simulink model "Forced_SMD_System"  (R2023b)
settings: Solver=VariableStepAuto  StartTime=0.0  StopTime=5  MaxStep=0.01  RelTol=1e-3
model workspace (MAT data in the model file):
  b = 0.5
  k = 1
  m = 10
settings Model: Creator=91839  LastModifiedBy=siva kumar
settings SolverCC: AlgebraicLoopSolver=TrustRegion
settings DataIOCC: ExternalInput=data  SaveFormat=Array  DSMLogging=off  ReturnWorkspaceOutputs=off
settings DebuggingCC: UnconnectedInputMsg=warning  UnconnectedOutputMsg=warning  UnconnectedLineMsg=warning
settings ModelReferenceCC: EnableRefExpFcnMdlSchedulingChecks=on
settings SFSimCC: CustomCodeUndefinedFunction=UseInterfaceOnly

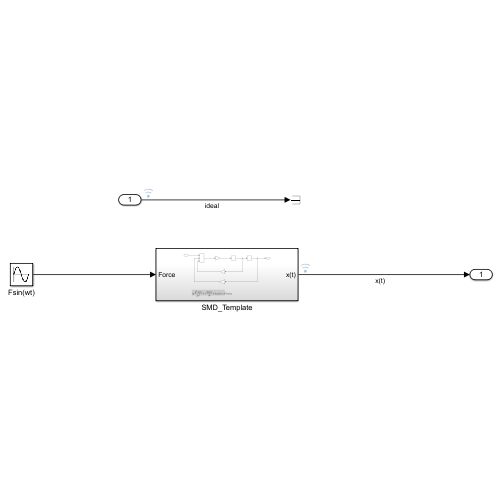
[thumbnail: Simulink's stored preview of the top-level diagram]
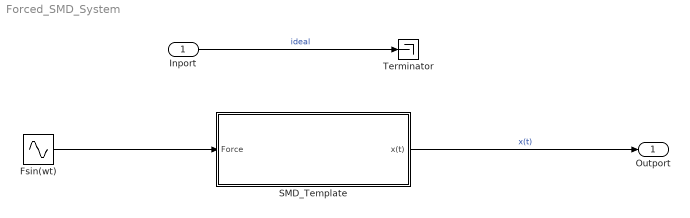
== system Forced_SMD_System ==
  Inport : Inport
  Fsin(wt) : Sin  Amplitude=100  Frequency=20  SampleTime=0
  SMD_Template : Subsystem
  Terminator : Terminator
  Outport : Outport
  wires:
  Inport/1 -> Terminator/1  "ideal"
  Fsin(wt)/1 -> SMD_Template/1(Force)
  SMD_Template/1(x(t)) -> Outport/1  "x(t)"

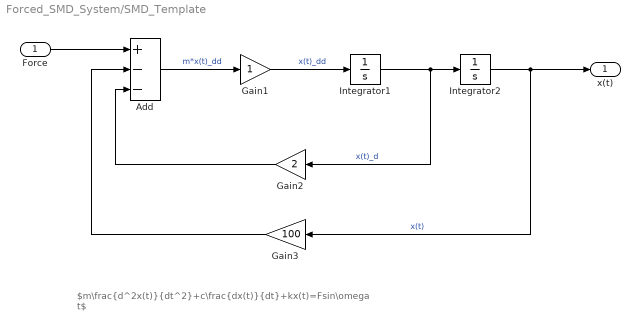
== system Forced_SMD_System/SMD_Template ==
  note: $m\frac{d^2x(t)}{dt^2}+c\frac{dx(t)}{dt}+kx(t)=Fsin\omega t$
  Force : Inport
  Add : Sum  Inputs=+--
  Gain1 : Gain
  Gain2 : Gain  Gain=2
  Gain3 : Gain  Gain=100
  Integrator1 : Integrator
  Integrator2 : Integrator  InitialCondition=0.02
  x(t) : Outport
  wires:
  Force/1 -> Add/1
  Add/1 -> Gain1/1  "m*x(t)_dd"
  Gain1/1 -> Integrator1/1  "x(t)_dd"
  Integrator1/1 -> Integrator2/1, Gain2/1  "x(t)_d"
  Integrator2/1 -> x(t)/1, Gain3/1  "x(t)"
  Gain2/1 -> Add/3
  Gain3/1 -> Add/2
